simulink model "FixedWing_Dynamic_Model_SIL_PX4"  (R2022b)
settings: Solver=ode4  StartTime=0.0  StopTime=inf  FixedStep=0.004  RelTol=1e-3
model workspace (MAT data in the model file):
  sample_time = 0.004
values from neighbouring files (symbols this model uses):
  uavData = struct    [InitFixedWingParam.m]
undefined symbols (not defined in the file or in its folder): Earth, env, WGS84
libraries: aerolibactuator x5, simulink_extras x3, aerolibasang x2, aerolibatmos2 x2, shared6dof x1, aerolibtransform2 x1, aerolibconvert2 x1, aerolibanimutils x1
(part 1 of 2)
settings Model: Creator=kboychev  LastModifiedBy=sergarro
settings OptimizationCC: ZeroExternalMemoryAtStartup=off  ZeroInternalMemoryAtStartup=off
settings ModelReferenceCC: EnableRefExpFcnMdlSchedulingChecks=on
settings RTWCC: Toolchain=Microsoft Visual C++ 2017 v15.0 | nmake (64-bit Windows)  TargetLang=C++
settings GRTTargetCC: TargetLangStandard=C++11 (ISO)  CodeInterfacePackaging=C++ class

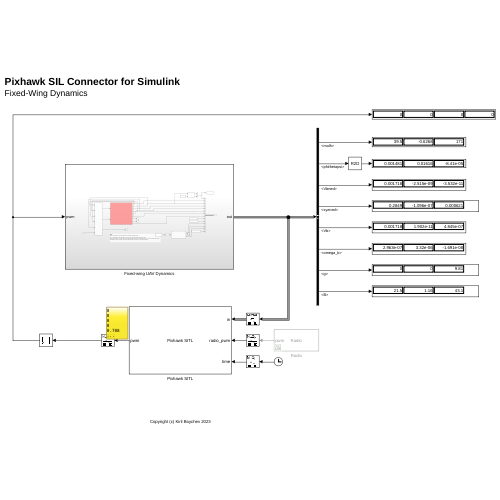
[thumbnail: Simulink's stored preview of the top-level diagram]
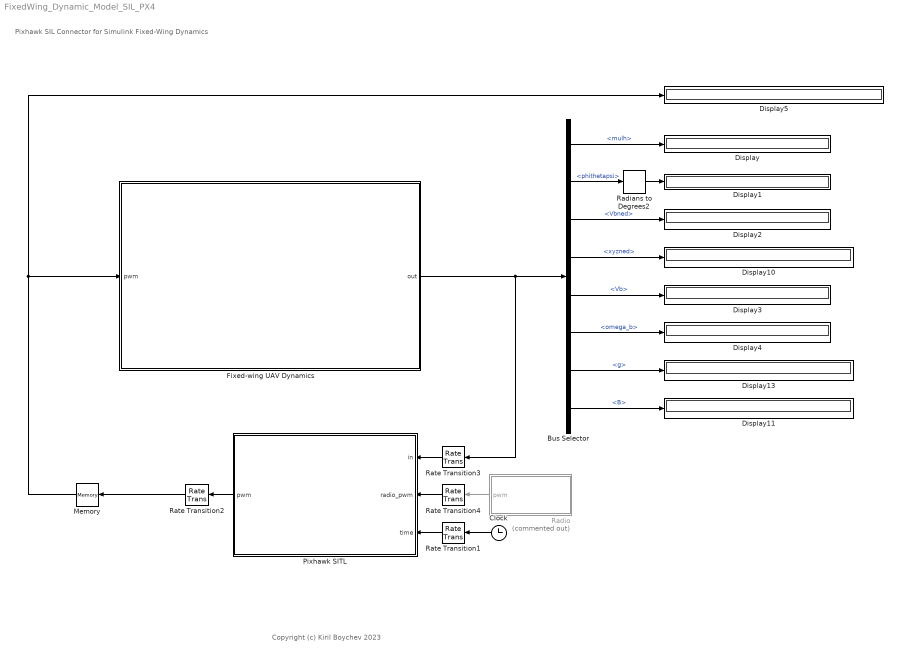
== system FixedWing_Dynamic_Model_SIL_PX4 ==
  note: Pixhawk SIL Connector for Simulink
      | Fixed-Wing Dynamics
  note: Copyright (c) Kiril Boychev 2023
  Bus Selector : BusSelector  OutputSignals=mulh,phithetapsi,Vbned,xyzned,Vb,omega_b,g,B
  Clock : Clock
  Display{,1..5,10..11,13} (9 alike) : Display
  Fixed-wing UAV Dynamics : Subsystem
  Memory : Memory  InitialCondition=[0 0 0 0]
  Pixhawk SITL : Subsystem
      mask Display:
      | fprintf('Pixhawk SITL');
      | port_label('input',1,'in');
      | port_label('input',2,'radio_pwm');
      | port_label('input',3,'time');
      | port_label('output',1,'pwm');
  Radians to Degrees2 : simulink_extras/Transformations/Radians to Degrees
  Radio : Subsystem  Commented=on
      mask Display:
      | fprintf('Radio');
      | port_label('output',1,'pwm');
  Rate Transition{1..4} (4 alike) : RateTransition  OutPortSampleTime=sample_time
  wires:
  Clock/1 -> Rate Transition1/1
  Radio/1(pwm) -> Rate Transition4/1
  Fixed-wing UAV Dynamics/1(out) -> Bus Selector/1, Rate Transition3/1
  Bus Selector/3 -> Display2/1  "<Vbned>"
  Bus Selector/1 -> Display/1  "<mulh>"
  Bus Selector/5 -> Display3/1  "<Vb>"
  Bus Selector/2 -> Radians to Degrees2/1  "<phithetapsi>"
  Bus Selector/8 -> Display11/1  "<B>"
  Radians to Degrees2/1 -> Display1/1
  Bus Selector/7 -> Display13/1  "<g>"
  Bus Selector/4 -> Display10/1  "<xyzned>"
  Bus Selector/6 -> Display4/1  "<omega_b>"
  Rate Transition2/1 -> Memory/1
  Pixhawk SITL/1(pwm) -> Rate Transition2/1
  Memory/1 -> Display5/1, Fixed-wing UAV Dynamics/1(pwm)
  Rate Transition3/1 -> Pixhawk SITL/1(in)
  Rate Transition1/1 -> Pixhawk SITL/3(time)
  Rate Transition4/1 -> Pixhawk SITL/2(radio_pwm)

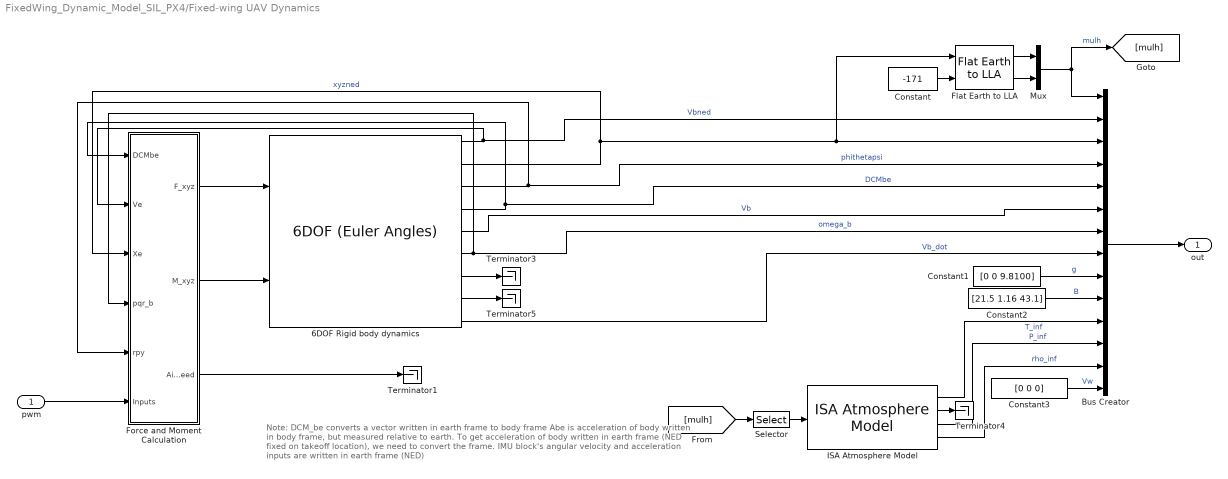
== system FixedWing_Dynamic_Model_SIL_PX4/Fixed-wing UAV Dynamics ==
  note: Note:
      | DCM_be converts a vector written in earth frame to body frame
      | Abe is acceleration of body written in body frame, but measured relative to earth.
      | To get acceleration of body written in earth frame (NED fixed on takeoff location), we need to convert the frame.
      | IMU block's angular velocity and acceleration inputs are written in earth frame (NED)
  pwm : Inport
  "6DOF Rigid body dynamics " : shared6dof/6DOF (Euler Angles)  units=Metric (MKS)  mtype=Fixed  rep=Quaternion  xme_0=init.posNED  Vm_0=init.vb  eul_0=init.euler  pm_0=init.angRates  mass_0=uavData.geometry.mass  mass_e=0.5  mass_f=2.0  inertia=diag([uavData.inertia.Ixx, uavData.inertia.Iyy, uavData.inertia.Izz])  inertia_e=eye(3)  inertia_f=2*eye(3)  k_quat=1  vre_flag=on  abi_flag=on  aMode=aMode  xme_statename=''  Vm_statename=''  eul_statename=''  quat_statename=''  pm_statename=''  mass_statename=''
  Bus Creator : BusCreator  Inputs=14
  Constant : Constant  Value=-171
  Constant1 : Constant  Value=[0 0 9.8100]
  Constant2 : Constant  Value=[21.5 1.16 43.1]
  Constant3 : Constant  Value=[0 0 0]
  Flat Earth to LLA : aerolibtransform2/Flat Earth to LLA  units=Metric (MKS)  ptype=Earth (WGS84)  F=1/298.257223563  R=6378137  refPosPort=off  LL0=[39.49738807491014, -0.6268122488722822]  psi=0
  Force and Moment Calculation : Subsystem
  ISA Atmosphere Model : aerolibatmos2/ISA Atmosphere Model  custom=off  g=9.80665  gamma=1.4  R=287.0531  L=0.0065  h_trop=11000  h_strat=20000  rho0=1.225  P0=101325  T0=288.15  h0=0
  Mux : Mux  Inputs=2
  Selector : Selector  IndexMode=Zero-based  InputPortWidth=3  IndexOptions=Index vector (dialog)  Indices=2  OutputSizes=1
  Terminator{1,3..5} (4 alike) : Terminator
  out : Outport
  wires:
  "6DOF Rigid body dynamics "/9 -> Bus Creator/8  "Vb_dot"
  Selector/1 -> ISA Atmosphere Model/1
  "6DOF Rigid body dynamics "/3 -> Bus Creator/4, Force and Moment Calculation/5(rpy)  "phithetapsi"
  Constant/1 -> Flat Earth to LLA/2
  Constant2/1 -> Bus Creator/10  "B"
  "6DOF Rigid body dynamics "/5 -> Bus Creator/6  "Vb"
  ISA Atmosphere Model/3 -> Bus Creator/12  "P_inf"
  ISA Atmosphere Model/2 -> Terminator4/1
  Bus Creator/1 -> out/1
  ISA Atmosphere Model/1 -> Bus Creator/11  "T_inf"
  "6DOF Rigid body dynamics "/4 -> Bus Creator/5, Force and Moment Calculation/1(DCMbe)  "DCMbe"
  "6DOF Rigid body dynamics "/6 -> Bus Creator/7, Force and Moment Calculation/4(pqr_b)  "omega_b"
  Force and Moment Calculation/1(F_xyz) -> "6DOF Rigid body dynamics "/1
  "6DOF Rigid body dynamics "/1 -> Bus Creator/2, Force and Moment Calculation/2(Ve)  "Vbned"
  Flat Earth to LLA/1 -> Mux/1
  Flat Earth to LLA/2 -> Mux/2
  Constant3/1 -> Bus Creator/14  "Vw"
  Force and Moment Calculation/2(M_xyz) -> "6DOF Rigid body dynamics "/2
  "6DOF Rigid body dynamics "/8 -> Terminator5/1
  [mulh] -> Selector/1
  "6DOF Rigid body dynamics "/7 -> Terminator3/1
  pwm/1 -> Force and Moment Calculation/6(Inputs)
  "6DOF Rigid body dynamics "/2 -> Flat Earth to LLA/1, Bus Creator/3, Force and Moment Calculation/3(Xe)  "xyzned"
  Force and Moment Calculation/3(Airspeed) -> Terminator1/1
  ISA Atmosphere Model/4 -> Bus Creator/13  "rho_inf"
  Mux/1 -> Bus Creator/1, [mulh]  "mulh"
  Constant1/1 -> Bus Creator/9  "g"

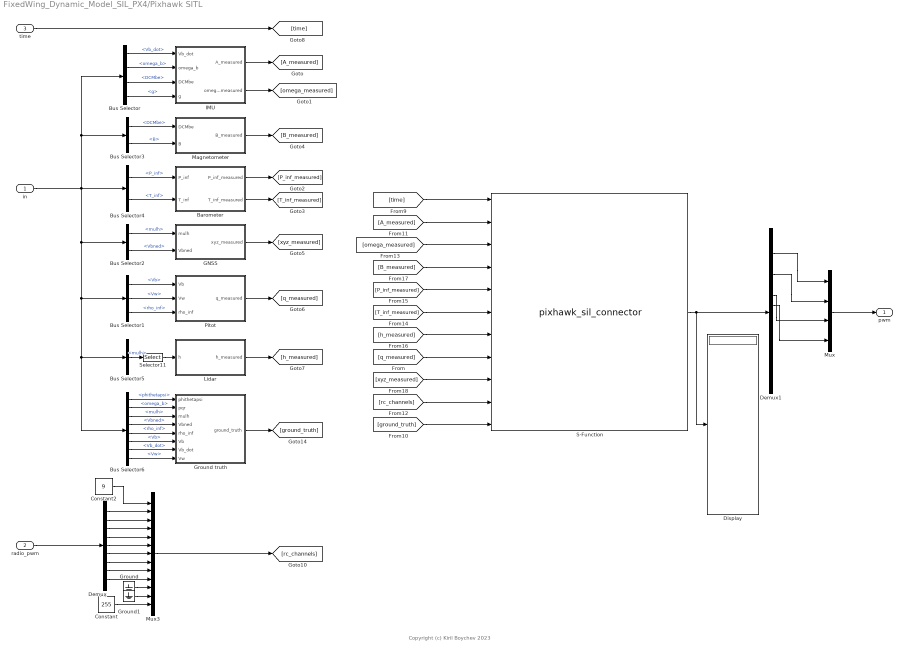
== system FixedWing_Dynamic_Model_SIL_PX4/Pixhawk SITL ==
  note: Copyright (c) Kiril Boychev 2023
  in : Inport
  radio_pwm : Inport  Port=2
  time : Inport  Port=3
  Barometer : Subsystem
  Bus Selector : BusSelector  OutputSignals=Vb_dot,omega_b,DCMbe,g
  Bus Selector1 : BusSelector  OutputSignals=Vb,Vw,rho_inf
  Bus Selector2 : BusSelector  OutputSignals=mulh,Vbned
  Bus Selector3 : BusSelector  OutputSignals=DCMbe,B
  Bus Selector4 : BusSelector  OutputSignals=P_inf,T_inf
  Bus Selector5 : BusSelector  OutputSignals=mulh
  Bus Selector6 : BusSelector  OutputSignals=phithetapsi,omega_b,mulh,Vbned,rho_inf,Vb,Vb_dot,Vw
  Constant : Constant  Value=255
  Constant2 : Constant  Value=9
  Demux : Demux  Outputs=9
  Demux1 : Demux  Outputs=16
  Display : Display
  GNSS : Subsystem
  Ground : Ground
  Ground truth : Subsystem
  Ground1 : Ground
  IMU : Subsystem
  Lidar : Subsystem
  Magnetometer : Subsystem
  Mux : Mux
  Mux3 : Mux  Inputs=13
  Pitot : Subsystem
  S-Function : S-Function  FunctionName=pixhawk_sil_connector  SFunctionDeploymentMode=off  EnableBusSupport=off
  Selector11 : Selector  IndexMode=Zero-based  InputPortWidth=3  IndexOptions=Index vector (dialog)  Indices=2  OutputSizes=1
  pwm : Outport
  wires:
  IMU/1(A_measured) -> [A_measured]
  IMU/2(omega_b_measured) -> [omega_measured]
  Bus Selector4/1 -> Barometer/1(P_inf)  "<P_inf>"
  Bus Selector4/2 -> Barometer/2(T_inf)  "<T_inf>"
  Barometer/1(P_inf_measured) -> [P_inf_measured]
  Barometer/2(T_inf_measured) -> [T_inf_measured]
  Magnetometer/1(B_measured) -> [B_measured]
  Bus Selector2/1 -> GNSS/1(mulh)  "<mulh>"
  Constant/1 -> Mux3/13
  Constant2/1 -> Mux3/1
  Demux/9 -> Mux3/10
  Demux/8 -> Mux3/9
  Demux/7 -> Mux3/8
  Demux/6 -> Mux3/7
  Demux/5 -> Mux3/6
  Demux/4 -> Mux3/5
  Demux/3 -> Mux3/4
  Demux/2 -> Mux3/3
  Demux/1 -> Mux3/2
  Ground truth/1(ground_truth) -> [ground_truth]
  Bus Selector3/1 -> Magnetometer/1(DCMbe)  "<DCMbe>"
  Bus Selector3/2 -> Magnetometer/2(B)  "<B>"
  Bus Selector/1 -> IMU/1(Vb_dot)  "<Vb_dot>"
  Bus Selector/3 -> IMU/3(DCMbe)  "<DCMbe>"
  Bus Selector/4 -> IMU/4(g)  "<g>"
  Bus Selector/2 -> IMU/2(omega_b)  "<omega_b>"
  GNSS/1(xyz_measured) -> [xyz_measured]
  radio_pwm/1 -> Demux/1
  Bus Selector2/2 -> GNSS/2(Vbned)  "<Vbned>"
  [time] -> S-Function/1
  [rc_channels] -> S-Function/10
  [A_measured] -> S-Function/2
  [B_measured] -> S-Function/4
  [T_inf_measured] -> S-Function/6
  [q_measured] -> S-Function/8
  [xyz_measured] -> S-Function/9
  [omega_measured] -> S-Function/3
  [P_inf_measured] -> S-Function/5
  [h_measured] -> S-Function/7
  [ground_truth] -> S-Function/11
  time/1 -> [time]
  Mux3/1 -> [rc_channels]
  Bus Selector1/3 -> Pitot/3(rho_inf)  "<rho_inf>"
  Bus Selector1/1 -> Pitot/1(Vb)  "<Vb>"
  in/1 -> Bus Selector4/1, Bus Selector/1, Bus Selector3/1, Bus Selector1/1, Bus Selector5/1, Bus Selector6/1, Bus Selector2/1
  Bus Selector1/2 -> Pitot/2(Vw)  "<Vw>"
  Pitot/1(q_measured) -> [q_measured]
  S-Function/1 -> Display/1, Demux1/1
  Bus Selector6/1 -> Ground truth/1(phithetapsi)  "<phithetapsi>"
  Bus Selector6/2 -> Ground truth/2(pqr)  "<omega_b>"
  Bus Selector6/8 -> Ground truth/8(Vw)  "<Vw>"
  Bus Selector6/7 -> Ground truth/7(Vb_dot)  "<Vb_dot>"
  Bus Selector6/6 -> Ground truth/6(Vb)  "<Vb>"
  Bus Selector6/5 -> Ground truth/5(rho_inf)  "<rho_inf>"
  Bus Selector6/4 -> Ground truth/4(Vbned)  "<Vbned>"
  Bus Selector6/3 -> Ground truth/3(mulh)  "<mulh>"
  Lidar/1(h_measured) -> [h_measured]
  Bus Selector5/1 -> Selector11/1  "<mulh>"
  Selector11/1 -> Lidar/1(h)
  Ground/1 -> Mux3/11
  Ground1/1 -> Mux3/12
  Mux/1 -> pwm/1
  Demux1/3 -> Mux/1
  Demux1/5 -> Mux/2
  Demux1/8 -> Mux/4
  Demux1/7 -> Mux/3

== system FixedWing_Dynamic_Model_SIL_PX4/Radio ==
  Mux : Mux  Inputs=9
  PWM Mapping : MATLAB Function  TreatAsAtomicUnit=on
  Pilot Joystick All : aerolibanimutils/Pilot Joystick  JoystickID=Joystick1  OutputConfiguration=AllOutputs  SampleTime=0.02
  Terminator : Terminator
  pwm : Outport
  wires:
  PWM Mapping/5(pwm5) -> Mux/5
  PWM Mapping/1(pwm1) -> Mux/1
  PWM Mapping/8(pwm8) -> Mux/8
  Mux/1 -> pwm/1
  PWM Mapping/7(pwm7) -> Mux/7
  PWM Mapping/9(pwm9) -> Mux/9
  PWM Mapping/3(pwm3) -> Mux/3
  PWM Mapping/4(pwm4) -> Mux/4
  PWM Mapping/6(pwm6) -> Mux/6
  PWM Mapping/2(pwm2) -> Mux/2
  Pilot Joystick All/3 -> Terminator/1
  Pilot Joystick All/2 -> PWM Mapping/2(buttons)
  Pilot Joystick All/1 -> PWM Mapping/1(analog)

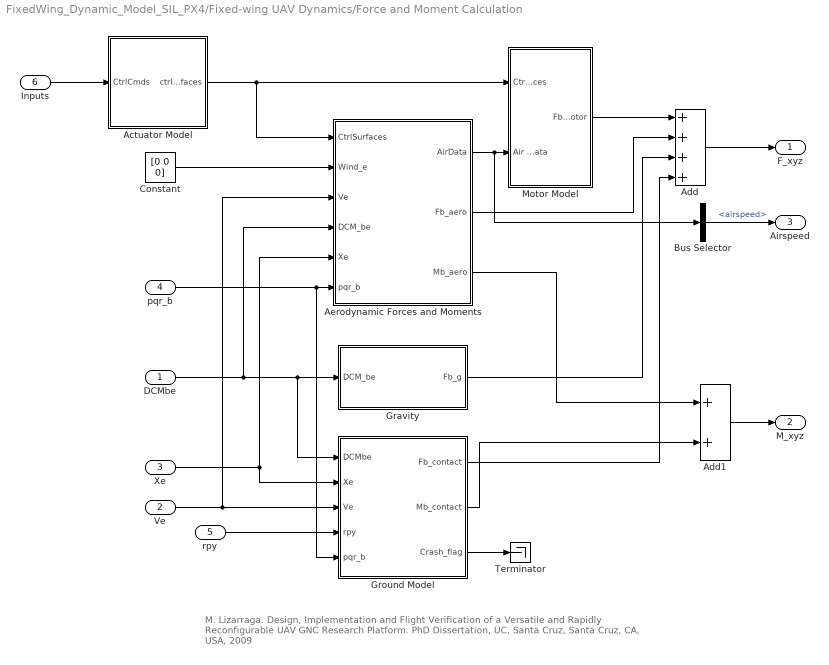
== system FixedWing_Dynamic_Model_SIL_PX4/Fixed-wing UAV Dynamics/Force and Moment Calculation ==
  note: M. Lizarraga. Design, Implementation and Flight Verification of a Versatile and Rapidly Reconfigurable UAV GNC Research Platform. PhD Dissertation, UC, Santa Cruz, Santa Cruz, CA, USA, 2009
  DCMbe : Inport
  Ve : Inport  Port=2
  Xe : Inport  Port=3
  pqr_b : Inport  Port=4
  rpy : Inport  Port=5
  Inputs : Inport  Port=6
  Actuator Model : Subsystem
  Add : Sum  Inputs=4
  Add1 : Sum  Inputs=2
  Aerodynamic Forces and Moments : Subsystem
  Bus Selector : BusSelector  OutputSignals=airspeed
  Constant : Constant  Value=[0 0 0]
  Gravity : Subsystem
  Ground Model : Subsystem
  Motor Model : Subsystem
  Terminator : Terminator
  F_xyz : Outport
  M_xyz : Outport  Port=2
  Airspeed : Outport  Port=3
  wires:
  Add/1 -> F_xyz/1
  DCMbe/1 -> Aerodynamic Forces and Moments/4(DCM_be), Ground Model/1(DCMbe), Gravity/1(DCM_be)
  pqr_b/1 -> Ground Model/5(pqr_b), Aerodynamic Forces and Moments/6(pqr_b)
  Actuator Model/1(ctrlSurfaces) -> Aerodynamic Forces and Moments/1(CtrlSurfaces), Motor Model/1(Ctrl Surfaces)
  Aerodynamic Forces and Moments/1(AirData) -> Bus Selector/1, Motor Model/2(Air Data)
  Ground Model/1(Fb_contact) -> Add/4
  Gravity/1(Fb_g) -> Add/3
  Motor Model/1(Fb_motor) -> Add/1
  Ve/1 -> Aerodynamic Forces and Moments/3(Ve), Ground Model/3(Ve)
  Ground Model/3(Crash_flag) -> Terminator/1
  Aerodynamic Forces and Moments/2(Fb_aero) -> Add/2
  Aerodynamic Forces and Moments/3(Mb_aero) -> Add1/1
  Xe/1 -> Aerodynamic Forces and Moments/5(Xe), Ground Model/2(Xe)
  Constant/1 -> Aerodynamic Forces and Moments/2(Wind_e)
  Inputs/1 -> Actuator Model/1(CtrlCmds)
  Bus Selector/1 -> Airspeed/1  "<airspeed>"
  rpy/1 -> Ground Model/4(rpy)
  Add1/1 -> M_xyz/1
  Ground Model/2(Mb_contact) -> Add1/2

== system FixedWing_Dynamic_Model_SIL_PX4/Pixhawk SITL/Barometer ==
  note: Copyright (c) Kiril Boychev 2023
  P_inf : Inport
  T_inf : Inport  Port=2
  Constant : Constant  Value=0.04
  Constant1 : Constant  Value=0.01
  K to degC : Bias  Bias=-273.15  SaturateOnIntegerOverflow=off
  Pa to hPa : Gain  Gain=0.01
  Product : Product
  Product1 : Product
  Random Number : RandomNumber  Seed=9  SampleTime=sample_time
  Random Number3 : RandomNumber  Seed=10  SampleTime=sample_time
  Sum1 : Sum  Inputs=++|
  Sum2 : Sum  Inputs=|++
  P_inf_measured : Outport
  T_inf_measured : Outport  Port=2
  wires:
  Sum1/1 -> Pa to hPa/1
  Random Number/1 -> Product/2
  Product/1 -> Sum1/1
  Constant/1 -> Product/1
  Sum2/1 -> T_inf_measured/1
  Random Number3/1 -> Product1/2
  Constant1/1 -> Product1/1
  Product1/1 -> Sum2/2
  T_inf/1 -> K to degC/1
  K to degC/1 -> Sum2/1
  P_inf/1 -> Sum1/2
  Pa to hPa/1 -> P_inf_measured/1

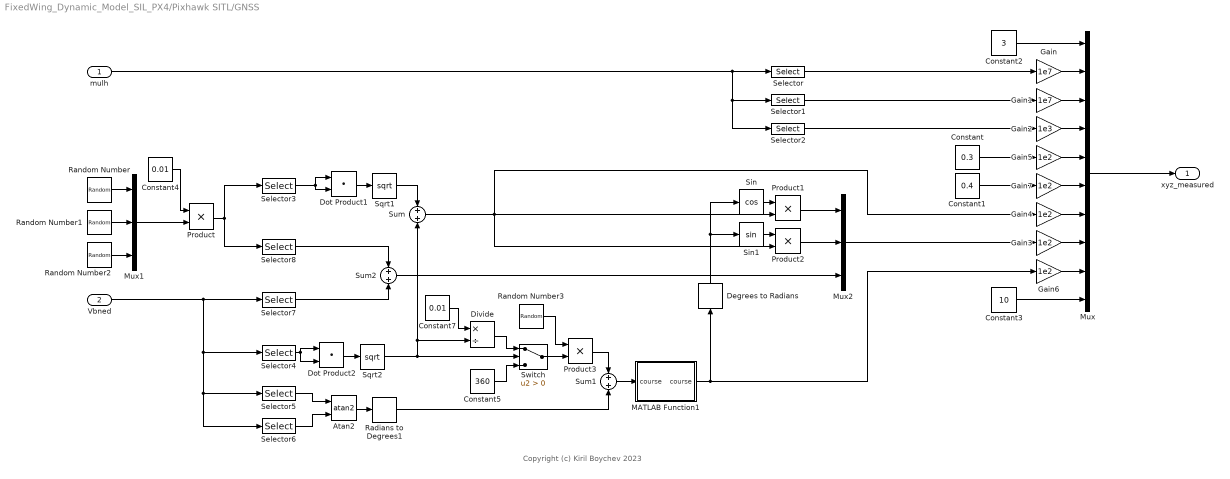
== system FixedWing_Dynamic_Model_SIL_PX4/Pixhawk SITL/GNSS ==
  note: Copyright (c) Kiril Boychev 2023
  mulh : Inport
  Vbned : Inport  Port=2
  Atan2 : Trigonometry  Operator=atan2
  Constant : Constant  Value=0.3
  Constant1 : Constant  Value=0.4
  Constant2 : Constant  Value=3
  Constant3 : Constant  Value=10
  Constant4 : Constant  Value=0.01
  Constant5 : Constant  Value=360
  Constant7 : Constant  Value=0.01
  Degrees to Radians : simulink_extras/Transformations/Degrees to Radians
  Divide : Product  Inputs=*/
  Dot Product1 : DotProduct  OutDataTypeStr=Inherit: Inherit via internal rule
  Dot Product2 : DotProduct  OutDataTypeStr=Inherit: Inherit via internal rule
  Gain : Gain  Gain=1e7
  Gain1 : Gain  Gain=1e7
  Gain2 : Gain  Gain=1e3
  Gain{3..7} (5 alike) : Gain  Gain=1e2
  MATLAB Function1 : MATLAB Function  TreatAsAtomicUnit=on
  Mux : Mux  Inputs=10
  Mux1 : Mux  Inputs=3
  Mux2 : Mux  Inputs=3
  Product{,1..3} (4 alike) : Product
  Radians to Degrees1 : simulink_extras/Transformations/Radians to Degrees
  Random Number : RandomNumber  Seed=11  SampleTime=sample_time
  Random Number1 : RandomNumber  Seed=12  SampleTime=sample_time
  Random Number2 : RandomNumber  Seed=13  SampleTime=sample_time
  Random Number3 : RandomNumber  Seed=14  SampleTime=sample_time
  Selector : Selector  IndexMode=Zero-based  InputPortWidth=3  IndexOptions=Index vector (dialog)  Indices=0  OutputSizes=1
  Selector1 : Selector  IndexMode=Zero-based  InputPortWidth=3  IndexOptions=Index vector (dialog)  Indices=1  OutputSizes=1
  Selector2 : Selector  IndexMode=Zero-based  InputPortWidth=3  IndexOptions=Index vector (dialog)  Indices=2  OutputSizes=1
  Selector3 : Selector  IndexMode=Zero-based  InputPortWidth=3  IndexOptions=Index vector (dialog)  Indices=[0 1]  OutputSizes=1
  Selector4 : Selector  IndexMode=Zero-based  InputPortWidth=3  IndexOptions=Index vector (dialog)  Indices=[0 1]  OutputSizes=1
  Selector5 : Selector  IndexMode=Zero-based  InputPortWidth=3  IndexOptions=Index vector (dialog)  Indices=1  OutputSizes=1
  Selector6 : Selector  IndexMode=Zero-based  InputPortWidth=3  IndexOptions=Index vector (dialog)  Indices=0  OutputSizes=1
  Selector7 : Selector  IndexMode=Zero-based  InputPortWidth=3  IndexOptions=Index vector (dialog)  Indices=2  OutputSizes=1
  Selector8 : Selector  IndexMode=Zero-based  InputPortWidth=3  IndexOptions=Index vector (dialog)  Indices=2  OutputSizes=1
  Sin : Trigonometry  Operator=cos
  Sin1 : Trigonometry
  Sqrt1 : Sqrt
  Sqrt2 : Sqrt
  Sum : Sum
  Sum1 : Sum
  Sum2 : Sum
  Switch : Switch  Criteria=u2 > Threshold  SaturateOnIntegerOverflow=off  InputSameDT=off
  xyz_measured : Outport
  wires:
  mulh/1 -> Selector1/1, Selector2/1, Selector/1
  Selector/1 -> Gain/1
  Selector1/1 -> Gain1/1
  Selector2/1 -> Gain2/1
  Constant2/1 -> Mux/1
  Gain/1 -> Mux/2
  Gain1/1 -> Mux/3
  Gain2/1 -> Mux/4
  Constant/1 -> Gain5/1
  Constant1/1 -> Gain7/1
  Gain4/1 -> Mux/7
  Gain3/1 -> Mux/8
  Gain6/1 -> Mux/9
  Constant3/1 -> Mux/10
  Mux/1 -> xyz_measured/1
  Gain5/1 -> Mux/5
  Gain7/1 -> Mux/6
  Selector5/1 -> Atan2/1
  Sum2/1 -> Mux2/3
  Random Number1/1 -> Mux1/2
  Mux1/1 -> Product/2
  Atan2/1 -> Radians to Degrees1/1
  Constant4/1 -> Product/1
  Selector3/1 -> Dot Product1/1, Dot Product1/2
  Product/1 -> Selector3/1, Selector8/1
  Random Number/1 -> Mux1/1
  Switch/1 -> Product3/2
  Sum/1 -> Product2/2, Gain4/1, Product1/2
  Constant7/1 -> Divide/1
  Sqrt2/1 -> Switch/2, Divide/2, Sum/2
  Random Number2/1 -> Mux1/3
  Selector4/1 -> Dot Product2/1, Dot Product2/2
  Dot Product1/1 -> Sqrt1/1
  Sin/1 -> Product1/1
  Random Number3/1 -> Product3/1
  Degrees to Radians/1 -> Sin/1, Sin1/1
  Divide/1 -> Switch/1
  Selector6/1 -> Atan2/2
  Sin1/1 -> Product2/1
  Sum1/1 -> MATLAB Function1/1("course ")
  Dot Product2/1 -> Sqrt2/1
  Radians to Degrees1/1 -> Sum1/2
  Product3/1 -> Sum1/1
  MATLAB Function1/1(course) -> Degrees to Radians/1, Gain6/1
  Constant5/1 -> Switch/3
  Product1/1 -> Mux2/1
  Product2/1 -> Mux2/2
  Mux2/1 -> Gain3/1
  Sqrt1/1 -> Sum/1
  Selector7/1 -> Sum2/2
  Selector8/1 -> Sum2/1
  Vbned/1 -> Selector6/1, Selector5/1, Selector4/1, Selector7/1

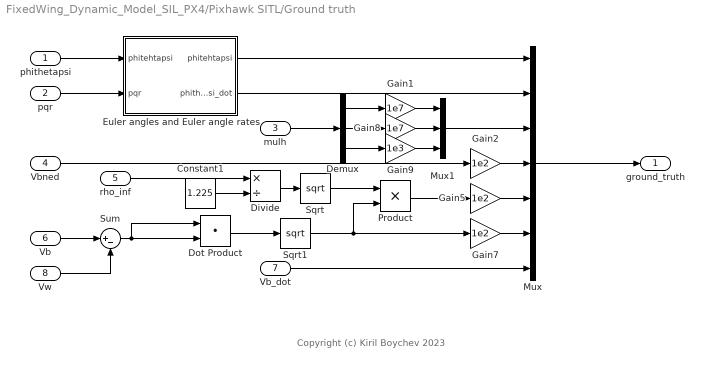
== system FixedWing_Dynamic_Model_SIL_PX4/Pixhawk SITL/Ground truth ==
  note: Copyright (c) Kiril Boychev 2023
  phithetapsi : Inport
  pqr : Inport  Port=2
  mulh : Inport  Port=3
  Vbned : Inport  Port=4
  rho_inf : Inport  Port=5
  Vb : Inport  Port=6
  Vb_dot : Inport  Port=7
  Vw : Inport  Port=8
  Constant1 : Constant  Value=1.225
  Demux : Demux  Outputs=3
  Divide : Product  Inputs=*/
  Dot Product : DotProduct  OutDataTypeStr=Inherit: Inherit via internal rule
  Euler angles and Euler angle rates : MATLAB Function  TreatAsAtomicUnit=on
  Gain1 : Gain  Gain=1e7
  Gain2 : Gain  Gain=1e2
  Gain5 : Gain  Gain=1e2
  Gain7 : Gain  Gain=1e2
  Gain8 : Gain  Gain=1e7
  Gain9 : Gain  Gain=1e3
  Mux : Mux  Inputs=7
  Mux1 : Mux  Inputs=3
  Product : Product
  Sqrt : Sqrt
  Sqrt1 : Sqrt
  Sum : Sum  Inputs=|+-
  ground_truth : Outport
  wires:
  Vbned/1 -> Gain2/1
  Mux/1 -> ground_truth/1
  Gain5/1 -> Mux/5
  Gain7/1 -> Mux/6
  mulh/1 -> Demux/1
  Demux/1 -> Gain1/1
  Demux/2 -> Gain8/1
  Demux/3 -> Gain9/1
  Gain1/1 -> Mux1/1
  Gain8/1 -> Mux1/2
  Gain9/1 -> Mux1/3
  Mux1/1 -> Mux/3
  Gain2/1 -> Mux/4
  Product/1 -> Gain5/1
  Vb_dot/1 -> Mux/7
  Euler angles and Euler angle rates/2(phithetapsi_dot) -> Mux/2
  Euler angles and Euler angle rates/1(phitehtapsi) -> Mux/1
  pqr/1 -> Euler angles and Euler angle rates/2(pqr)
  phithetapsi/1 -> Euler angles and Euler angle rates/1("phitehtapsi ")
  Sqrt1/1 -> Gain7/1, Product/2
  Sum/1 -> Dot Product/1, Dot Product/2
  Divide/1 -> Sqrt/1
  Constant1/1 -> Divide/2
  rho_inf/1 -> Divide/1
  Sqrt/1 -> Product/1
  Dot Product/1 -> Sqrt1/1
  Vb/1 -> Sum/1
  Vw/1 -> Sum/2

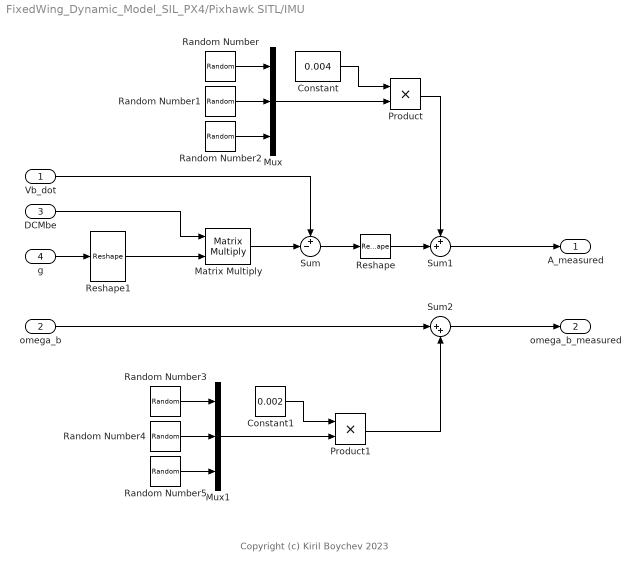
== system FixedWing_Dynamic_Model_SIL_PX4/Pixhawk SITL/IMU ==
  note: Copyright (c) Kiril Boychev 2023
  Vb_dot : Inport
  omega_b : Inport  Port=2
  DCMbe : Inport  Port=3
  g : Inport  Port=4
  Constant : Constant  Value=0.004
  Constant1 : Constant  Value=0.002
  Matrix Multiply : Product  Multiplication=Matrix(*)
  Mux : Mux  Inputs=3
  Mux1 : Mux  Inputs=3
  Product : Product
  Product1 : Product
  Random Number : RandomNumber  SampleTime=sample_time
  Random Number1 : RandomNumber  Seed=1  SampleTime=sample_time
  Random Number2 : RandomNumber  Seed=2  SampleTime=sample_time
  Random Number3 : RandomNumber  Seed=3  SampleTime=sample_time
  Random Number4 : RandomNumber  Seed=4  SampleTime=sample_time
  Random Number5 : RandomNumber  Seed=5  SampleTime=sample_time
  Reshape : Reshape
  Reshape1 : Reshape  OutputDimensionality=Column vector (2-D)
  Sum : Sum  Inputs=+-|
  Sum1 : Sum  Inputs=++|
  Sum2 : Sum  Inputs=|++
  A_measured : Outport
  omega_b_measured : Outport  Port=2
  wires:
  g/1 -> Reshape1/1
  DCMbe/1 -> Matrix Multiply/1
  Matrix Multiply/1 -> Sum/2
  Vb_dot/1 -> Sum/1
  Reshape1/1 -> Matrix Multiply/2
  Sum/1 -> Reshape/1
  Sum1/1 -> A_measured/1
  Random Number1/1 -> Mux/2
  Random Number/1 -> Mux/1
  Random Number2/1 -> Mux/3
  Mux/1 -> Product/2
  Product/1 -> Sum1/1
  Constant/1 -> Product/1
  Sum2/1 -> omega_b_measured/1
  Mux1/1 -> Product1/2
  Random Number4/1 -> Mux1/2
  Random Number3/1 -> Mux1/1
  Random Number5/1 -> Mux1/3
  Constant1/1 -> Product1/1
  Product1/1 -> Sum2/2
  omega_b/1 -> Sum2/1
  Reshape/1 -> Sum1/2

== system FixedWing_Dynamic_Model_SIL_PX4/Pixhawk SITL/Lidar ==
  note: Copyright (c) Kiril Boychev 2023
  h : Inport
  Bias : Bias  Bias=-488  SaturateOnIntegerOverflow=off
  Constant1 : Constant  Value=0.005
  Product2 : Product
  Random Number1 : RandomNumber  Seed=16  SampleTime=sample_time
  Sum3 : Sum  Inputs=|++
  m to cm : Gain  Gain=1e2
  h_measured : Outport
  wires:
  Constant1/1 -> Product2/1
  Product2/1 -> Sum3/2
  Random Number1/1 -> Product2/2
  h/1 -> Bias/1
  Bias/1 -> Sum3/1
  Sum3/1 -> m to cm/1
  m to cm/1 -> h_measured/1

== system FixedWing_Dynamic_Model_SIL_PX4/Pixhawk SITL/Magnetometer ==
  note: Copyright (c) Kiril Boychev 2023
  DCMbe : Inport
  B : Inport  Port=2
  Constant : Constant  Value=0.01
  Matrix Multiply : Product  Multiplication=Matrix(*)
  Mux : Mux  Inputs=3
  Product : Product
  Random Number : RandomNumber  Seed=6  SampleTime=sample_time
  Random Number1 : RandomNumber  Seed=7  SampleTime=sample_time
  Random Number2 : RandomNumber  Seed=8  SampleTime=sample_time
  Sum1 : Sum  Inputs=++|
  uT to Gauss : Gain  Gain=0.0100
  B_measured : Outport
  wires:
  Product/1 -> Sum1/1
  Random Number1/1 -> Mux/2
  Mux/1 -> Product/2
  Random Number/1 -> Mux/1
  Constant/1 -> Product/1
  Random Number2/1 -> Mux/3
  Matrix Multiply/1 -> Sum1/2
  DCMbe/1 -> Matrix Multiply/1
  Sum1/1 -> uT to Gauss/1
  B/1 -> Matrix Multiply/2
  uT to Gauss/1 -> B_measured/1

== system FixedWing_Dynamic_Model_SIL_PX4/Pixhawk SITL/Pitot ==
  note: Copyright (c) Kiril Boychev 2023
  Vb : Inport
  Vw : Inport  Port=2
  rho_inf : Inport  Port=3
  Constant : Constant  Value=0.5
  Constant1 : Constant  Value=0.01
  Pa to hPa : Gain  Gain=0.01
  Product : Product  Inputs=3
  Product1 : Product
  Random Number3 : RandomNumber  Seed=15  SampleTime=sample_time
  Selector : Selector  IndexMode=Zero-based  InputPortWidth=3  IndexOptions=Index vector (dialog)  Indices=0  OutputSizes=1
  Square1 : Math  Operator=square
  Sum : Sum  Inputs=++|
  Sum1 : Sum  Inputs=|+-
  q_measured : Outport
  wires:
  Product1/1 -> Sum/1
  Random Number3/1 -> Product1/2
  Constant1/1 -> Product1/1
  Pa to hPa/1 -> Sum/2
  Sum/1 -> q_measured/1
  Selector/1 -> Square1/1
  Square1/1 -> Product/1
  rho_inf/1 -> Product/2
  Constant/1 -> Product/3
  Product/1 -> Pa to hPa/1
  Vw/1 -> Sum1/2
  Vb/1 -> Sum1/1
  Sum1/1 -> Selector/1

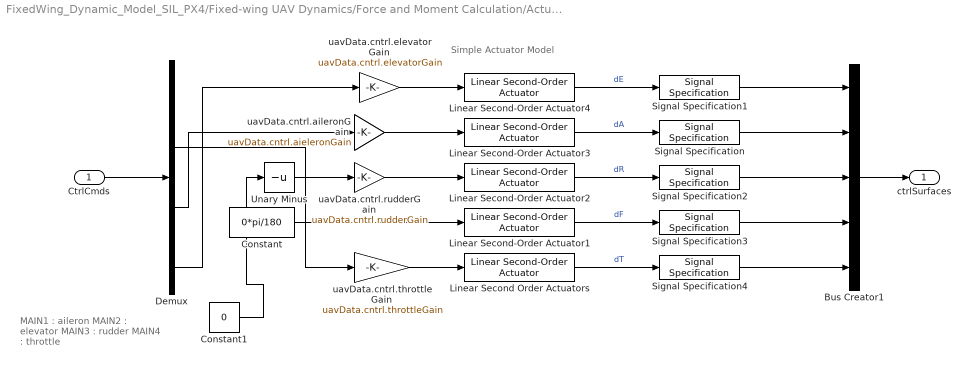
== system FixedWing_Dynamic_Model_SIL_PX4/Fixed-wing UAV Dynamics/Force and Moment Calculation/Actuator Model ==
  note: Simple Actuator Model
  note: MAIN1 : aileron
      | MAIN2 : elevator
      | MAIN3 : rudder
      | MAIN4 : throttle
  CtrlCmds : Inport
  Bus Creator1 : BusCreator  Inputs=5
  Constant : Constant  Value=0*pi/180
  Constant1 : Constant  Value=0
  Demux : Demux
  Linear Second Order Actuators : aerolibactuator/Linear Second-Order Actuator  wn_fin=35  z_fin=0.75  fin_act_0=0  fin_act_vel=0
      settings: AttributesFormatString=|
      | Nat Freq => %<wn_fin>
      | Damping => %<z_fin>
  Linear Second-Order Actuator{1..4} (4 alike) : aerolibactuator/Linear Second-Order Actuator  wn_fin=35  z_fin=0.75  fin_act_0=0  fin_act_vel=0
  Signal Specification{,1..3} (4 alike) : SignalSpecification  Unit=rad
  Signal Specification4 : SignalSpecification  Unit=%
  Unary Minus : UnaryMinus
  uavData.cntrl.aileronGain : Gain  Gain=uavData.cntrl.aieleronGain
  uavData.cntrl.elevatorGain : Gain  Gain=uavData.cntrl.elevatorGain
  uavData.cntrl.rudderGain : Gain  Gain=uavData.cntrl.rudderGain
  uavData.cntrl.throttleGain : Gain  Gain=uavData.cntrl.throttleGain
  ctrlSurfaces : Outport  VectorParamsAs1DForOutWhenUnconnected=off
  wires:
  uavData.cntrl.elevatorGain/1 -> Linear Second-Order Actuator4/1
  uavData.cntrl.aileronGain/1 -> Linear Second-Order Actuator3/1
  uavData.cntrl.rudderGain/1 -> Linear Second-Order Actuator2/1
  Constant/1 -> Linear Second-Order Actuator1/1
  uavData.cntrl.throttleGain/1 -> Linear Second Order Actuators/1
  Bus Creator1/1 -> ctrlSurfaces/1
  Linear Second-Order Actuator4/1 -> Signal Specification1/1  "dE"
  Linear Second-Order Actuator3/1 -> Signal Specification/1  "dA"
  Linear Second-Order Actuator2/1 -> Signal Specification2/1  "dR"
  Linear Second-Order Actuator1/1 -> Signal Specification3/1  "dF"
  Linear Second Order Actuators/1 -> Signal Specification4/1  "dT"
  CtrlCmds/1 -> Demux/1
  Signal Specification1/1 -> Bus Creator1/1
  Signal Specification/1 -> Bus Creator1/2
  Signal Specification2/1 -> Bus Creator1/3
  Signal Specification3/1 -> Bus Creator1/4
  Signal Specification4/1 -> Bus Creator1/5
  Unary Minus/1 -> uavData.cntrl.rudderGain/1
  Demux/2 -> uavData.cntrl.throttleGain/1
  Constant1/1 -> Unary Minus/1
  Demux/4 -> uavData.cntrl.elevatorGain/1
  Demux/3 -> uavData.cntrl.aileronGain/1

== system FixedWing_Dynamic_Model_SIL_PX4/Fixed-wing UAV Dynamics/Force and Moment Calculation/Aerodynamic Forces and Moments ==
  CtrlSurfaces : Inport
  Wind_e : Inport  Port=2
  Ve : Inport  Port=3
  DCM_be : Inport  Port=4
  Xe : Inport  Port=5
  pqr_b : Inport  Port=6
  Compute Air Data : Subsystem  TreatAsAtomicUnit=on  VariantControl=use_aerospace_blocks == 1
  Compute Body Frame Forces and Moments : Subsystem
  Compute Rho : Subsystem
  Rotate Vw : Subsystem
  Vair : Sum  Inputs=+-  InputSameDT=on  SaturateOnIntegerOverflow=on  OutDataTypeStr=Inherit: Same as first input
  AirData : Outport  VectorParamsAs1DForOutWhenUnconnected=off
  Fb_aero : Outport  Port=2
  Mb_aero : Outport  Port=3
  wires:
  Ve/1 -> Vair/1
  Compute Body Frame Forces and Moments/1(F_b) -> Fb_aero/1
  Wind_e/1 -> Vair/2
  CtrlSurfaces/1 -> Compute Body Frame Forces and Moments/2(CtrlSurfaces)
  Compute Air Data/1(AirData) -> Compute Body Frame Forces and Moments/1(AirData), AirData/1
  Compute Body Frame Forces and Moments/2(M_b) -> Mb_aero/1
  Rotate Vw/1(Vb) -> Compute Air Data/1(Vb)
  Compute Rho/1(Rho) -> Compute Air Data/2(Rho)
  Vair/1 -> Rotate Vw/1(Vw)
  pqr_b/1 -> Compute Body Frame Forces and Moments/3(p,q,r)
  DCM_be/1 -> Rotate Vw/2(DCM_be)
  Xe/1 -> Compute Rho/1(Xe)

== system FixedWing_Dynamic_Model_SIL_PX4/Fixed-wing UAV Dynamics/Force and Moment Calculation/Gravity ==
  DCM_be : Inport
  Constant : Constant  Value=[0 0 env.ISA_g]'
  Gain : Gain  Gain=uavData.geometry.mass
  Matrix Multiply : Product  Multiplication=Matrix(*)
  Fb_g : Outport
  wires:
  Matrix Multiply/1 -> Gain/1
  Constant/1 -> Matrix Multiply/2
  DCM_be/1 -> Matrix Multiply/1
  Gain/1 -> Fb_g/1

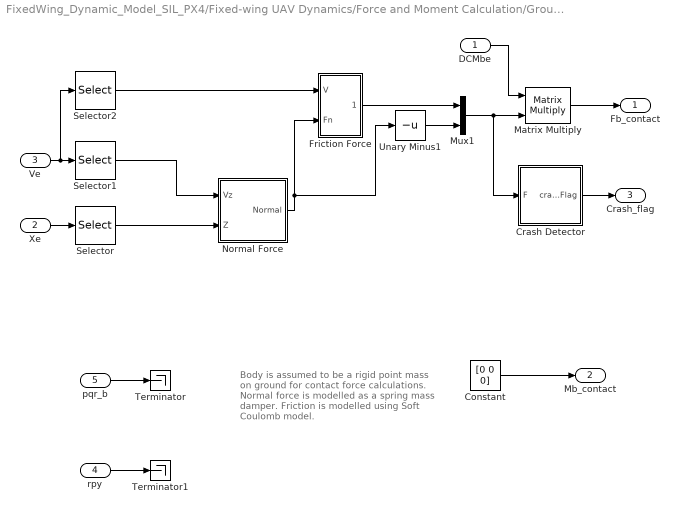
== system FixedWing_Dynamic_Model_SIL_PX4/Fixed-wing UAV Dynamics/Force and Moment Calculation/Ground Model ==
  note: Body is assumed to be a rigid point mass on ground for contact force calculations.
      |
      | Normal force is modelled as a spring mass damper.
      |
      | Friction is modelled using Soft Coulomb model.
  DCMbe : Inport
  Xe : Inport  Port=2
  Ve : Inport  Port=3
  rpy : Inport  Port=4
  pqr_b : Inport  Port=5
  Constant : Constant  Value=[0 0 0]
  Crash Detector : Subsystem
  Friction Force : Subsystem
  Matrix Multiply : Product  Multiplication=Matrix(*)
  Mux1 : Mux  Inputs=2
  Normal Force : Subsystem
  Selector : Selector  InputPortWidth=3  IndexOptions=Index vector (dialog)  Indices=[3]  OutputSizes=1
  Selector1 : Selector  InputPortWidth=3  IndexOptions=Index vector (dialog)  Indices=[3]  OutputSizes=1
  Selector2 : Selector  InputPortWidth=3  IndexOptions=Index vector (dialog)  Indices=[1,2]  OutputSizes=1
  Terminator : Terminator
  Terminator1 : Terminator
  Unary Minus1 : UnaryMinus
  Fb_contact : Outport
  Mb_contact : Outport  Port=2
  Crash_flag : Outport  Port=3
  wires:
  Crash Detector/1(crashFlag) -> Crash_flag/1
  Xe/1 -> Selector/1
  Ve/1 -> Selector2/1, Selector1/1
  Selector1/1 -> Normal Force/1(Vz)
  Selector/1 -> Normal Force/2(Z)
  DCMbe/1 -> Matrix Multiply/1
  Matrix Multiply/1 -> Fb_contact/1
  Normal Force/1(Normal) -> Friction Force/2(Fn), Unary Minus1/1
  Mux1/1 -> Matrix Multiply/2, Crash Detector/1(F)
  Unary Minus1/1 -> Mux1/2
  Selector2/1 -> Friction Force/1(V)
  Friction Force/1(Friction) -> Mux1/1
  pqr_b/1 -> Terminator/1
  rpy/1 -> Terminator1/1
  Constant/1 -> Mb_contact/1

== system FixedWing_Dynamic_Model_SIL_PX4/Fixed-wing UAV Dynamics/Force and Moment Calculation/Motor Model ==
  Ctrl Surfaces : Inport
  Air Data : Inport  Port=2
  Bus Selector : BusSelector  OutputSignals=dT
  Bus Selector1 : BusSelector  OutputSignals=airspeed
  Engine Model : Subsystem
  Fb_motor : Outport  VectorParamsAs1DForOutWhenUnconnected=off
  wires:
  Bus Selector1/1 -> Engine Model/2(Airspeed)  "<airspeed>"
  Ctrl Surfaces/1 -> Bus Selector/1
  Air Data/1 -> Bus Selector1/1
  Bus Selector/1 -> Engine Model/1(dt)  "<dT>"
  Engine Model/1(Thrust_b) -> Fb_motor/1

== system FixedWing_Dynamic_Model_SIL_PX4/Fixed-wing UAV Dynamics/Force and Moment Calculation/Aerodynamic Forces and Moments/Compute Air Data ==
  Vb : Inport  PortDimensions=3
  Rho : Inport  Port=2
  Bus Creator : BusCreator  Inputs=4
  Demux : Demux  Outputs=3
  Dynamic Pressure : aerolibasang/Dynamic Pressure
  Subsystem : Subsystem
  AirData : Outport  VectorParamsAs1DForOutWhenUnconnected=off
  wires:
  Bus Creator/1 -> AirData/1
  Rho/1 -> Dynamic Pressure/2
  Dynamic Pressure/1 -> Bus Creator/4  "q"
  Vb/1 -> Subsystem/1(Vb), Dynamic Pressure/1
  Subsystem/1(airData) -> Demux/1
  Demux/1 -> Bus Creator/1  "alpha"
  Demux/2 -> Bus Creator/2  "beta"
  Demux/3 -> Bus Creator/3  "airspeed"

== system FixedWing_Dynamic_Model_SIL_PX4/Fixed-wing UAV Dynamics/Force and Moment Calculation/Aerodynamic Forces and Moments/Compute Body Frame Forces and Moments ==
  AirData : Inport
  CtrlSurfaces : Inport  Port=2
  p,q,r : Inport  Port=3
  Bus Selector : BusSelector  OutputSignals=alpha,beta
  Mux : Mux  Inputs=2
  Rotate FM to body frame : Subsystem
  Wind frame F& M : Subsystem
  F_b : Outport  Unit=kg*m/s^2  VectorParamsAs1DForOutWhenUnconnected=off
  M_b : Outport  Port=2  Unit=N*m  VectorParamsAs1DForOutWhenUnconnected=off
  wires:
  Mux/1 -> Rotate FM to body frame/2(alpha_beta)
  Bus Selector/2 -> Mux/2  "<beta>"
  Bus Selector/1 -> Mux/1  "<alpha>"
  Wind frame F& M/1(FM_w) -> Rotate FM to body frame/1(FM_w)  "FM_W"
  p,q,r/1 -> Wind frame F& M/3(p,q,r)
  Rotate FM to body frame/2(M_b) -> M_b/1
  Rotate FM to body frame/1(F_b) -> F_b/1
  CtrlSurfaces/1 -> Wind frame F& M/2(CtrlSurfaces)
  AirData/1 -> Wind frame F& M/1(Airdata), Bus Selector/1

== system FixedWing_Dynamic_Model_SIL_PX4/Fixed-wing UAV Dynamics/Force and Moment Calculation/Aerodynamic Forces and Moments/Compute Rho ==
  Xe : Inport
  Gain : Gain  Gain=-1
      settings: AttributesFormatString=Z to Alt
  Get Z : Selector  InputPortWidth=3  IndexOptions=Index vector (dialog)  Indices=[3]  OutputSizes=[(-2)]
  ISA Atmosphere Model1 : aerolibatmos2/ISA Atmosphere Model  custom=on  g=env.ISA_g  gamma=1.4  R=env.ISA_R  L=env.ISA_lapse  h_trop=11000  h_strat=20000  rho0=env.ISA_rho0  P0=env.ISA_P0  T0=env.ISA_T0  h0=0
  Terminator : Terminator
  Terminator1 : Terminator
  Terminator2 : Terminator
  Transfer Fcn : TransferFcn  Denominator=[.01 1]
  Rho : Outport  VectorParamsAs1DForOutWhenUnconnected=off
  wires:
  ISA Atmosphere Model1/2 -> Terminator1/1
  ISA Atmosphere Model1/1 -> Terminator/1  "OAT"
  Gain/1 -> ISA Atmosphere Model1/1
  Get Z/1 -> Transfer Fcn/1
  Transfer Fcn/1 -> Gain/1
  ISA Atmosphere Model1/3 -> Terminator2/1  "static"
  Xe/1 -> Get Z/1
  ISA Atmosphere Model1/4 -> Rho/1

== system FixedWing_Dynamic_Model_SIL_PX4/Fixed-wing UAV Dynamics/Force and Moment Calculation/Aerodynamic Forces and Moments/Rotate Vw ==
  Vw : Inport
  DCM_be : Inport  Port=2
  RL2B * Vw : Product  Multiplication=Matrix(*)  InputSameDT=on  SaturateOnIntegerOverflow=on  OutDataTypeStr=Inherit: Same as first input
  Vb : Outport  Unit=m/s  VectorParamsAs1DForOutWhenUnconnected=off
  wires:
  RL2B * Vw/1 -> Vb/1
  Vw/1 -> RL2B * Vw/2
  DCM_be/1 -> RL2B * Vw/1

== system FixedWing_Dynamic_Model_SIL_PX4/Fixed-wing UAV Dynamics/Force and Moment Calculation/Ground Model/Crash Detector ==
  F : Inport
  Constant : Constant  Value=true
  Constant1 : Constant  Value=false
  Gain : Gain  Gain=1/(env.ISA_g*uavData.geometry.mass)
  Switch : Switch  Criteria=u2 > Threshold  Threshold=uavData.contact.gLimit  SaturateOnIntegerOverflow=off  InputSameDT=off
  norm1 : Subsystem
  crashFlag : Outport
  wires:
  F/1 -> norm1/1(F)
  norm1/1(Out1) -> Gain/1
  Switch/1 -> crashFlag/1
  Constant/1 -> Switch/1
  Constant1/1 -> Switch/3
  Gain/1 -> Switch/2

== system FixedWing_Dynamic_Model_SIL_PX4/Fixed-wing UAV Dynamics/Force and Moment Calculation/Ground Model/Friction Force ==
  V : Inport
  Fn : Inport  Port=2
  Product : Product
  Soft Coulomb Friction : Subsystem
  Unary Minus : UnaryMinus
  Friction : Outport
  wires:
  Fn/1 -> Product/2
  Soft Coulomb Friction/1(Out1) -> Product/1
  Product/1 -> Unary Minus/1
  Unary Minus/1 -> Friction/1
  V/1 -> Soft Coulomb Friction/1(V)

== system FixedWing_Dynamic_Model_SIL_PX4/Fixed-wing UAV Dynamics/Force and Moment Calculation/Ground Model/Normal Force ==
  Vz : Inport
  Z : Inport  Port=2
  Add : Sum
  Constant : Constant  Value=0
  Damper : Gain  Gain=-uavData.contact.damper
  Saturation : Saturate  UpperLimit=inf  LowerLimit=0
  Spring Kp : Gain  Gain=-uavData.contact.spring
  Switch : Switch  Criteria=u2 > Threshold  SaturateOnIntegerOverflow=off  InputSameDT=off
  Unary Minus : UnaryMinus
  Unary Minus1 : UnaryMinus
  Normal : Outport
  wires:
  Constant/1 -> Switch/1
  Z/1 -> Unary Minus/1
  Switch/1 -> Saturation/1
  Damper/1 -> Add/2
  Add/1 -> Switch/3
  Spring Kp/1 -> Add/1
  Vz/1 -> Unary Minus1/1
  Saturation/1 -> Normal/1
  Unary Minus/1 -> Spring Kp/1, Switch/2
  Unary Minus1/1 -> Damper/1

== system FixedWing_Dynamic_Model_SIL_PX4/Fixed-wing UAV Dynamics/Force and Moment Calculation/Motor Model/Engine Model ==
  dt : Inport
  Airspeed : Inport  Port=2
  Constant4 : Constant  Value=0
      settings: AttributesFormatString=%<Value>
  Get To : Subsystem
  Mass Conversion : aerolibconvert2/Mass Conversion  IU=lbm  OU=kg
  Mux : Mux  Inputs=2
  Mux1 : Mux  Inputs=3
  Saturation : Saturate  UpperLimit=inf  LowerLimit=0
  Thrust Available (lbs) : Fcn  Expr=u(1) - 0.047*sqrt(u(1))*u(2)
  kg2N : Gain  Gain=env.ISA_g  SaturateOnIntegerOverflow=on  OutDataTypeStr=Inherit: Same as input  ParamDataTypeStr=Inherit: Same as input
      settings: AttributesFormatString=%<Gain>
  Thrust_b : Outport  Unit=kg*m/s^2  VectorParamsAs1DForOutWhenUnconnected=off
  wires:
  Constant4/1 -> Mux1/3, Mux1/2
  Mass Conversion/1 -> kg2N/1
  Mux1/1 -> Thrust_b/1
  Airspeed/1 -> Mux/2
  Thrust Available (lbs)/1 -> Mass Conversion/1
  Mux/1 -> Thrust Available (lbs)/1
  Get To/1(To) -> Mux/1
  dt/1 -> Get To/1(dt)
  kg2N/1 -> Saturation/1
  Saturation/1 -> Mux1/1

== system FixedWing_Dynamic_Model_SIL_PX4/Fixed-wing UAV Dynamics/Force and Moment Calculation/Aerodynamic Forces and Moments/Compute Air Data/Subsystem ==
  note: Avoid singularity at low speeds
  Vb : Inport
  "Incidence, Sideslip, & Airspeed" : aerolibasang/Incidence, Sideslip, & Airspeed
  Mux : Mux  Inputs=3
  Mux1 : Mux  Inputs=3
  Switch : Switch  Criteria=u2 > Threshold  Threshold=0.1  SaturateOnIntegerOverflow=off  InputSameDT=off
  alpha : Constant  Value=0
  beta : Constant  Value=0
  norm : Subsystem
  airData : Outport
  wires:
  "Incidence, Sideslip, & Airspeed"/1 -> Mux/1  "alpha"
  "Incidence, Sideslip, & Airspeed"/3 -> Mux/3  "airspeed"
  Vb/1 -> norm/1(In1), "Incidence, Sideslip, & Airspeed"/1
  norm/1(Out1) -> Mux1/3, Switch/2
  "Incidence, Sideslip, & Airspeed"/2 -> Mux/2  "beta"
  Switch/1 -> airData/1
  Mux/1 -> Switch/1
  alpha/1 -> Mux1/1
  beta/1 -> Mux1/2
  Mux1/1 -> Switch/3

== system FixedWing_Dynamic_Model_SIL_PX4/Fixed-wing UAV Dynamics/Force and Moment Calculation/Aerodynamic Forces and Moments/Compute Body Frame Forces and Moments/Rotate FM to body frame ==
  FM_w : Inport
  alpha_beta : Inport  Port=2
  Forces : Selector  InputPortWidth=6  IndexOptions=Index vector (dialog)  Indices=[1 2 3]  OutputSizes=[(-2)]
  Moments : Selector  InputPortWidth=6  IndexOptions=Index vector (dialog)  Indices=[4 5 6]  OutputSizes=[(-2)]
  Rotate Forces : Subsystem
  Rotate Moments : Subsystem
  F_b : Outport  VectorParamsAs1DForOutWhenUnconnected=off
  M_b : Outport  Port=2  VectorParamsAs1DForOutWhenUnconnected=off
  wires:
  alpha_beta/1 -> Rotate Forces/2(alpha_beta), Rotate Moments/1(alpha_beta)
  Moments/1 -> Rotate Moments/2(M_w)
  FM_w/1 -> Forces/1, Moments/1
  Forces/1 -> Rotate Forces/1(F_w)
  Rotate Moments/1(M_b) -> M_b/1
  Rotate Forces/1(F_b) -> F_b/1

== system FixedWing_Dynamic_Model_SIL_PX4/Fixed-wing UAV Dynamics/Force and Moment Calculation/Aerodynamic Forces and Moments/Compute Body Frame Forces and Moments/Wind frame F& M ==
  Airdata : Inport
  CtrlSurfaces : Inport  Port=2
  p,q,r : Inport  Port=3
  Bus Creator1 : BusCreator  Inputs=2
  Bus Selector1 : BusSelector  OutputSignals=dA,dR
  Bus Selector2 : BusSelector  OutputSignals=dE,dF
  Bus Selector6 : BusSelector  OutputSignals=beta,airspeed
  Bus Selector7 : BusSelector  OutputSignals=alpha,airspeed
  Get Forces and Moments : Subsystem
  Lateral Channel : Subsystem
  Longitudinal Channel : Subsystem
  FM_w : Outport  PortDimensions=6  VectorParamsAs1DForOutWhenUnconnected=off
  wires:
  Get Forces and Moments/1(FM_w) -> FM_w/1
  Bus Creator1/1 -> Get Forces and Moments/2(AeroCoeffs)
  Bus Selector7/2 -> Longitudinal Channel/2(Airpseed)  "<airspeed>"
  Bus Selector7/1 -> Longitudinal Channel/1(alpha)  "<alpha>"
  Bus Selector6/2 -> Lateral Channel/2(Airspeed)  "<airspeed>"
  Bus Selector6/1 -> Lateral Channel/1(beta)  "<beta>"
  Airdata/1 -> Bus Selector6/1, Bus Selector7/1, Get Forces and Moments/1(Airdata)
  Bus Selector2/2 -> Longitudinal Channel/4(dF)  "<dF>"
  Bus Selector2/1 -> Longitudinal Channel/3(dE)  "<dE>"
  Bus Selector1/2 -> Lateral Channel/4(dR)  "<dR>"
  Bus Selector1/1 -> Lateral Channel/3(dA)  "<dA>"
  CtrlSurfaces/1 -> Bus Selector1/1, Bus Selector2/1
  p,q,r/1 -> Lateral Channel/5(p,q,r), Longitudinal Channel/5(p,q,r)
  Lateral Channel/1(Lateral) -> Bus Creator1/1
  Longitudinal Channel/1(Longitudinal) -> Bus Creator1/2

== system FixedWing_Dynamic_Model_SIL_PX4/Fixed-wing UAV Dynamics/Force and Moment Calculation/Ground Model/Crash Detector/norm1 ==
  F : Inport
  Dot Product : DotProduct  OutDataTypeStr=Inherit: Inherit via internal rule
  Sqrt : Sqrt
  Out1 : Outport
  wires:
  Dot Product/1 -> Sqrt/1
  F/1 -> Dot Product/2, Dot Product/1
  Sqrt/1 -> Out1/1

== system FixedWing_Dynamic_Model_SIL_PX4/Fixed-wing UAV Dynamics/Force and Moment Calculation/Ground Model/Friction Force/Soft Coulomb Friction ==
  note: Pennestrì, E., Rossi, V., Salvini, P. et al. Review and comparison of dry friction force models. Nonlinear Dyn 83, 1785–1801 (2016). https://doi.org/10.1007/s11071-015-2485-3
  V : Inport
  Tanh : Trigonometry  Operator=tanh
  friction coefficient : Gain  Gain=uavData.contact.rollingFriction
  vd : Gain  Gain=1/uavData.contact.vd
  Out1 : Outport
  wires:
  V/1 -> vd/1
  vd/1 -> Tanh/1
  Tanh/1 -> friction coefficient/1
  friction coefficient/1 -> Out1/1

== system FixedWing_Dynamic_Model_SIL_PX4/Fixed-wing UAV Dynamics/Force and Moment Calculation/Motor Model/Engine Model/Get To ==
  dt : Inport
  Divide : Product  Inputs=3
  Math Function : Math  Operator=pow  SignedPower=on
  Math Function1 : Math  Operator=pow  SignedPower=on
  MaxRPM : Gain  Gain=7200  SaturateOnIntegerOverflow=on  OutDataTypeStr=Inherit: Same as input  ParamDataTypeStr=Inherit: Same as input
      settings: AttributesFormatString=%<Gain>
  MaxRPM1 : Gain  Gain=uavData.engine.TFact  SaturateOnIntegerOverflow=on  OutDataTypeStr=Inherit: Same as input  ParamDataTypeStr=Inherit: Same as input
      settings: AttributesFormatString=%<Gain>
  Min RPM : Constant  Value=2000
      settings: AttributesFormatString=%<Value>
  Min Th K : Constant  Value=uavData.engine.MinThK
      settings: AttributesFormatString=%<Value>
  Prop Diameter (in) : Constant  Value=17
      settings: AttributesFormatString=%<Value>
  Prop Diameter (in)1 : Constant  Value=2
      settings: AttributesFormatString=%<Value>
  Prop Diameter (in)2 : Constant  Value=4
      settings: AttributesFormatString=%<Value>
  Saturation : Saturate  UpperLimit=1.0  LowerLimit=0
      settings: AttributesFormatString="[%<LowerLimit>  %<UpperLimit>]"
  Sum : Sum  Inputs=|++
  Sum1 : Sum  Inputs=|++
  Th K : Gain  Gain=uavData.engine.ThK  SaturateOnIntegerOverflow=on  OutDataTypeStr=Inherit: Same as input  ParamDataTypeStr=Inherit: Same as input
      settings: AttributesFormatString=%<Gain>
  To Constant : Constant  Value=2.83e-12
      settings: AttributesFormatString=%<Value>
  To : Outport  VectorParamsAs1DForOutWhenUnconnected=off
  wires:
  Min Th K/1 -> Sum1/2
  Sum1/1 -> MaxRPM/1
  dt/1 -> Saturation/1
  Th K/1 -> Sum1/1
  MaxRPM/1 -> Sum/1
  Min RPM/1 -> Sum/2
  Sum/1 -> Math Function/1
  MaxRPM1/1 -> To/1
  Divide/1 -> MaxRPM1/1
  To Constant/1 -> Divide/3
  Math Function1/1 -> Divide/2
  Math Function/1 -> Divide/1
  Prop Diameter (in)/1 -> Math Function1/1
  Prop Diameter (in)2/1 -> Math Function1/2
  Prop Diameter (in)1/1 -> Math Function/2
  Saturation/1 -> Th K/1

== system FixedWing_Dynamic_Model_SIL_PX4/Fixed-wing UAV Dynamics/Force and Moment Calculation/Aerodynamic Forces and Moments/Compute Air Data/Subsystem/norm ==
  In1 : Inport
  Dot Product : DotProduct  OutDataTypeStr=Inherit: Inherit via internal rule
  Sqrt : Sqrt
  Out1 : Outport
  wires:
  In1/1 -> Dot Product/2, Dot Product/1
  Dot Product/1 -> Sqrt/1
  Sqrt/1 -> Out1/1

== system FixedWing_Dynamic_Model_SIL_PX4/Fixed-wing UAV Dynamics/Force and Moment Calculation/Aerodynamic Forces and Moments/Compute Body Frame Forces and Moments/Rotate FM to body frame/Rotate Forces ==
  F_w : Inport
  alpha_beta : Inport  Port=2
  Product2 : Product  Multiplication=Matrix(*)  SaturateOnIntegerOverflow=on  OutDataTypeStr=Inherit: Same as first input
  RB2W : Subsystem
  RW2B : Math  Operator=transpose  SignedPower=on
  F_b : Outport  PortDimensions=3  VectorParamsAs1DForOutWhenUnconnected=off
  wires:
  RW2B/1 -> Product2/1
  F_w/1 -> Product2/2
  Product2/1 -> F_b/1
  alpha_beta/1 -> RB2W/1(aoa beta)
  RB2W/1(Rw2b) -> RW2B/1

== system FixedWing_Dynamic_Model_SIL_PX4/Fixed-wing UAV Dynamics/Force and Moment Calculation/Aerodynamic Forces and Moments/Compute Body Frame Forces and Moments/Rotate FM to body frame/Rotate Moments ==
  alpha_beta : Inport
  M_w : Inport  Port=2
  Matrix Multiply : Product  Multiplication=Matrix(*)
  RB2W : Subsystem
  RW2B : Math  Operator=transpose  SignedPower=on
  M_b : Outport  PortDimensions=3  VectorParamsAs1DForOutWhenUnconnected=off
  wires:
  RB2W/1(Rw2b) -> RW2B/1
  alpha_beta/1 -> RB2W/1(aoa beta)
  M_w/1 -> Matrix Multiply/2
  RW2B/1 -> Matrix Multiply/1
  Matrix Multiply/1 -> M_b/1

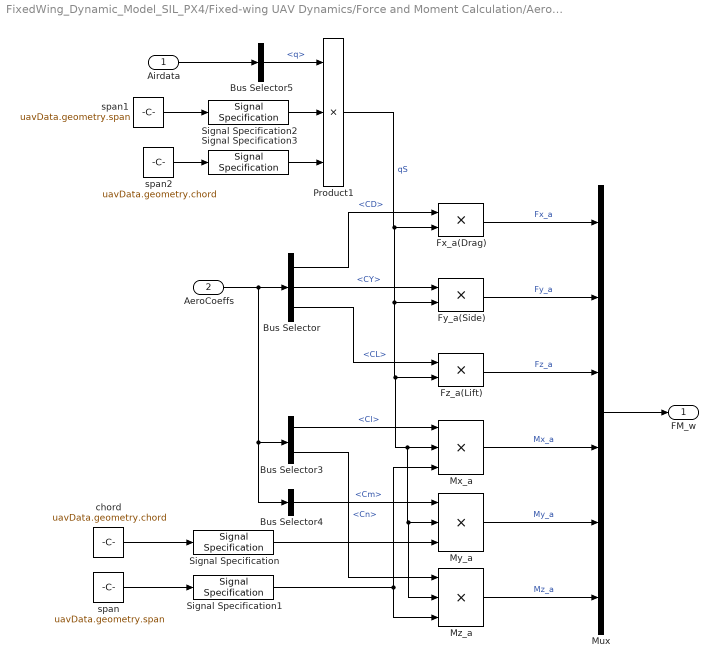
== system FixedWing_Dynamic_Model_SIL_PX4/Fixed-wing UAV Dynamics/Force and Moment Calculation/Aerodynamic Forces and Moments/Compute Body Frame Forces and Moments/Wind frame F& M/Get Forces and Moments ==
  Airdata : Inport
  AeroCoeffs : Inport  Port=2
  Bus Selector : BusSelector  OutputSignals=signal2.CD,signal1.CY,signal2.CL
  Bus Selector3 : BusSelector  OutputSignals=signal1.Cl,signal1.Cn
  Bus Selector4 : BusSelector  OutputSignals=signal2.Cm
  Bus Selector5 : BusSelector  OutputSignals=q
  Fx_a(Drag) : Product  Inputs=**  SaturateOnIntegerOverflow=on  OutDataTypeStr=Inherit: Same as first input
  Fy_a(Side) : Product  SaturateOnIntegerOverflow=on  OutDataTypeStr=Inherit: Same as first input
  Fz_a(Lift) : Product  SaturateOnIntegerOverflow=on  OutDataTypeStr=Inherit: Same as first input
  Mux : Mux  Inputs=6
  Mx_a : Product  Inputs=3  SaturateOnIntegerOverflow=on  OutDataTypeStr=Inherit: Same as first input
  My_a : Product  Inputs=3  SaturateOnIntegerOverflow=on  OutDataTypeStr=Inherit: Same as first input
  Mz_a : Product  Inputs=3  SaturateOnIntegerOverflow=on  OutDataTypeStr=Inherit: Same as first input
  Product1 : Product  Inputs=3  SaturateOnIntegerOverflow=on  OutDataTypeStr=Inherit: Same as first input
  Signal Specification{,1..3} (4 alike) : SignalSpecification  Unit=m
  chord : Constant  Value=uavData.geometry.chord  VectorParams1D=off
      settings: AttributesFormatString=%<Value>
  span : Constant  Value=uavData.geometry.span  VectorParams1D=off
      settings: AttributesFormatString=%<Value>
  span1 : Constant  Value=uavData.geometry.span  VectorParams1D=off
      settings: AttributesFormatString=%<Value>
  span2 : Constant  Value=uavData.geometry.chord  VectorParams1D=off
      settings: AttributesFormatString=%<Value>
  FM_w : Outport  VectorParamsAs1DForOutWhenUnconnected=off
  wires:
  Mx_a/1 -> Mux/4  "Mx_a"
  Bus Selector/2 -> Fy_a(Side)/1  "<CY>"
  Bus Selector4/1 -> My_a/1  "<Cm>"
  span2/1 -> Signal Specification3/1
  Fx_a(Drag)/1 -> Mux/1  "Fx_a"
  Bus Selector/1 -> Fx_a(Drag)/1  "<CD>"
  AeroCoeffs/1 -> Bus Selector/1, Bus Selector4/1, Bus Selector3/1
  My_a/1 -> Mux/5  "My_a"
  Fz_a(Lift)/1 -> Mux/3  "Fz_a"
  Mz_a/1 -> Mux/6  "Mz_a"
  Airdata/1 -> Bus Selector5/1
  chord/1 -> Signal Specification/1
  span/1 -> Signal Specification1/1
  Fy_a(Side)/1 -> Mux/2  "Fy_a"
  Mux/1 -> FM_w/1
  Bus Selector3/2 -> Mz_a/1  "<Cn>"
  Bus Selector/3 -> Fz_a(Lift)/1  "<CL>"
  Product1/1 -> Fx_a(Drag)/2, Fy_a(Side)/2, Fz_a(Lift)/2, Mx_a/2, My_a/2, Mz_a/2  "qS"
  span1/1 -> Signal Specification2/1
  Bus Selector3/1 -> Mx_a/1  "<Cl>"
  Bus Selector5/1 -> Product1/1  "<q>"
  Signal Specification/1 -> My_a/3
  Signal Specification1/1 -> Mz_a/3, Mx_a/3
  Signal Specification2/1 -> Product1/2
  Signal Specification3/1 -> Product1/3

== system FixedWing_Dynamic_Model_SIL_PX4/Fixed-wing UAV Dynamics/Force and Moment Calculation/Aerodynamic Forces and Moments/Compute Body Frame Forces and Moments/Wind frame F& M/Lateral Channel ==
  beta : Inport
  Airspeed : Inport  Port=2
  dA : Inport  Port=3
  dR : Inport  Port=4
  p,q,r : Inport  Port=5
  Bus Creator : BusCreator  Inputs=3
  CY : Subsystem
  Cl : Subsystem
  Cn : Subsystem
  Lateral : Outport  VectorParamsAs1DForOutWhenUnconnected=off
  wires:
  Cl/1(Cl) -> Bus Creator/2  "Cl"
  p,q,r/1 -> Cn/4(p,q,r), Cl/4(p,q,r)
  Airspeed/1 -> Cn/5(Airspeed), Cl/5(Airspeed)
  dR/1 -> CY/2(dR), Cl/3(dR), Cn/3(Dr)
  dA/1 -> Cl/2(dA), Cn/2(dA)
  beta/1 -> CY/1(beta), Cl/1(beta), Cn/1(beta)
  Cn/1(Cn) -> Bus Creator/3  "Cn"
  CY/1(CY) -> Bus Creator/1  "CY"
  Bus Creator/1 -> Lateral/1

== system FixedWing_Dynamic_Model_SIL_PX4/Fixed-wing UAV Dynamics/Force and Moment Calculation/Aerodynamic Forces and Moments/Compute Body Frame Forces and Moments/Wind frame F& M/Longitudinal Channel ==
  alpha : Inport
  Airpseed : Inport  Port=2
  dE : Inport  Port=3
  dF : Inport  Port=4
  p,q,r : Inport  Port=5
  Bus Creator : BusCreator  Inputs=3
  CD : Subsystem
  CL : Subsystem
  Cm : Subsystem
  Transfer Fcn : TransferFcn  Numerator=[1 0]  Denominator=[0.1 1]
  Y-down : Gain  Gain=-1  SaturateOnIntegerOverflow=on  OutDataTypeStr=Inherit: Same as input  ParamDataTypeStr=Inherit: Same as input
      settings: AttributesFormatString=%<Gain>
  Longitudinal : Outport  VectorParamsAs1DForOutWhenUnconnected=off
  wires:
  Transfer Fcn/1 -> CL/2(alpha_dot)
  Airpseed/1 -> CL/6(Airspeed)
  p,q,r/1 -> Cm/4(p,q,r), CL/5(p,q,r)
  dF/1 -> Cm/3(Df), CL/4(dF)
  Bus Creator/1 -> Longitudinal/1
  Cm/1(Cm) -> Bus Creator/3  "Cm"
  CL/1(CL) -> CD/1(CL), Y-down/1
  dE/1 -> Cm/2(De), CL/3(dE)
  Y-down/1 -> Bus Creator/2  "CL"
  CD/1(CD) -> Bus Creator/1  "CD"
  alpha/1 -> Transfer Fcn/1, Cm/1(alpha), CL/1(alpha)

== system FixedWing_Dynamic_Model_SIL_PX4/Fixed-wing UAV Dynamics/Force and Moment Calculation/Aerodynamic Forces and Moments/Compute Body Frame Forces and Moments/Rotate FM to body frame/Rotate Forces/RB2W ==
  aoa beta : Inport
  11 : Fcn  Expr=u[3]*u[4]
  12 : Fcn  Expr=u[2]
  13 : Fcn  Expr=u[1]*u[4]
  21 : Fcn  Expr=-u[3]*u[2]
  22 : Fcn  Expr=u[4]
  23 : Fcn  Expr=-u[1]*u[2]
  31 : Fcn  Expr=-u[1]
  32 : Fcn  Expr=0
  33 : Fcn  Expr=u[3]
  Mux : Mux  Inputs=2
  Mux3 : Mux  Inputs=9
  Reshape 9x1->3x3 : Reshape  OutputDimensionality=Customize  OutputDimensions=[3,3]
  sincos : Trigonometry  Operator=sincos
  Rw2b : Outport  VectorParamsAs1DForOutWhenUnconnected=off
  wires:
  Mux/1 -> 11/1, 21/1, 31/1, 12/1, 22/1, 32/1, 13/1, 23/1, 33/1
  aoa beta/1 -> sincos/1
  sincos/2 -> Mux/2
  sincos/1 -> Mux/1
  33/1 -> Mux3/9
  23/1 -> Mux3/8
  13/1 -> Mux3/7
  32/1 -> Mux3/6
  22/1 -> Mux3/5
  12/1 -> Mux3/4
  31/1 -> Mux3/3
  21/1 -> Mux3/2
  11/1 -> Mux3/1
  Reshape 9x1->3x3/1 -> Rw2b/1
  Mux3/1 -> Reshape 9x1->3x3/1
